simulink model "ACSwt_DD"  (R2016b)
settings: configuration reference "CodeGenConfigSet" (kept outside this file)
values from neighbouring files (symbols this model uses):
  AirC_tiSwtDebHiLo_C = Calibration.Parameter    [init_ACSwt_DD.m]    (also in init_ACSwt_DD_SIL.m = Simulink.Parameter)
  AirC_tiSwtDebLoHi_C = Calibration.Parameter    [init_ACSwt_DD.m]    (also in init_ACSwt_DD_SIL.m = Simulink.Parameter)
undefined symbols (not defined in the file or in its folder): ACSwt_DD_DT
libraries: CXLib x1
settings Model: Creator=胡炎林  LastModifiedBy=lenovo
settings ConfigSetRef: SourceLocation=Base Workspace

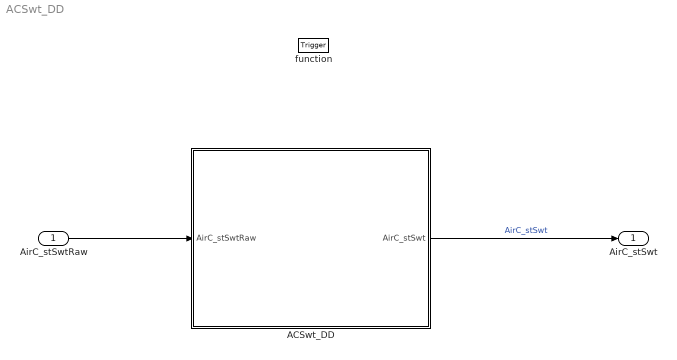
== system ACSwt_DD ==
  AirC_stSwtRaw : Inport  Description=Raw value of AC-switch read from the sensor  OutMin=0  OutMax=1  OutDataTypeStr=boolean
  function : TriggerPort  TriggerType=function-call  VariantControl=Variant
  ACSwt_DD : Subsystem
  AirC_stSwt : Outport  Description=Status of AC switch  OutMin=0  OutMax=1  OutDataTypeStr=boolean
  wires:
  ACSwt_DD/1(AirC_stSwt) -> AirC_stSwt/1  "AirC_stSwt"
  AirC_stSwtRaw/1 -> ACSwt_DD/1(AirC_stSwtRaw)

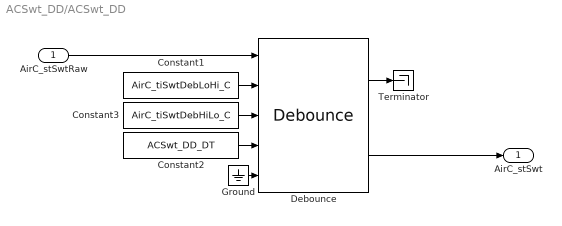
== system ACSwt_DD/ACSwt_DD ==
  AirC_stSwtRaw : Inport  Description=Raw value of AC-switch read from the sensor  OutMin=0  OutMax=1  OutDataTypeStr=boolean
  Constant1 : Constant  Value=AirC_tiSwtDebLoHi_C
  Constant2 : Constant  Value=ACSwt_DD_DT
  Constant3 : Constant  Value=AirC_tiSwtDebHiLo_C
  Debounce : CXLib/Debounce
  Ground : Ground
  Terminator : Terminator
  AirC_stSwt : Outport
  wires:
  Debounce/1 -> Terminator/1
  Constant1/1 -> Debounce/2
  Ground/1 -> Debounce/5
  Constant2/1 -> Debounce/4
  Constant3/1 -> Debounce/3
  Debounce/2 -> AirC_stSwt/1
  AirC_stSwtRaw/1 -> Debounce/1
